simulink library "Utilities"  (R2020b)
settings: Solver=VariableStepAuto  StartTime=0.0  StopTime=10.0  RelTol=1e-3

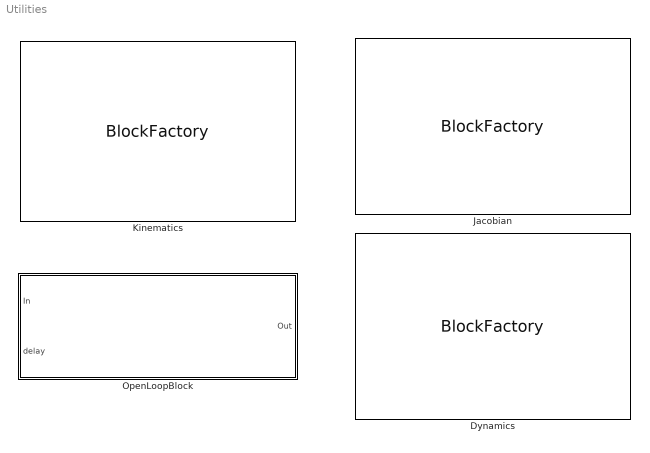
== system Utilities ==
  Dynamics : S-Function  FunctionName=BlockFactory  Parameters='XBotBlock_Dynamics','Dynamics',ModelName,ComponentsList  SFunctionDeploymentMode=off  EnableBusSupport=off  mask{ModelName=DefaultModel, ComponentsList={ 'B', 'BInv', 'M', 'H', 'tau_g', 'tau_id', 'tau_id_const' }}
  Jacobian : S-Function  FunctionName=BlockFactory  Parameters='XBotBlock_Jacobian','Jacobian',ModelName,JacobianList,LinkName,TargetFrame,ExternalRef,TargetLink,BaseLink  SFunctionDeploymentMode=off  EnableBusSupport=off  mask{ModelName=DefaultModel, JacobianList={ 'J', 'J_postural', 'J_relative', 'J_COM', 'dJcomQdot', 'JdotQdot', 'JdotQdot_relative' }, LinkName=, TargetFrame=, ExternalRef=Off, TargetLink=, BaseLink=}
      mask init:
      | mask_params = Simulink.Mask.get(gcb);
      | link_frame_param= mask_params.Parameters(3);
      | target_frame_param = mask_params.Parameters(4);
      | ext_ref_param = mask_params.Parameters(5);
      | target_link_param= mask_params.Parameters(6);
      | base_link_param = mask_params.Parameters(7);
      | 
      | 
      | set_enabled=false;
      | if(~bdIsLibrary(bdroot))
      |     model_status=get_param(bdroot,'SimulationStatus');
      |     if(model_status=="stopped")
      |         set_enabled=true;
      |     end
      | else
      |     set_enabled=true;
      | end
      | 
      | if(set_enabled)
      |     link_frame_param.set('Enabled','off'); 
      |     target_frame_param.set('Enabled','off');  
      |     ext_ref_param.set('Enabled','off');  
      |     target_link_param.set('Enabled','off');   
      |     base_link_param.set('Enabled','off');   
      | 
      | 
      |     %Get Number of input and output ports.
      |     portHandles = get_param(gcb,'PortHandles');
      |     %Input ports
      |     inputPorts=length(portHandles.Inport);
      |     %Output ports
      |     outputPorts=length(portHandles.Outport);
      | 
      | 
      |     % Get block mask handle
      |     maskObj = Simulink.Mask.get(gcb); 
      | 
      |     % Readings Selected
      |     itemsSelected=maskObj.getParameter('JacobianList').Value;
      |     itemsSelected=regexprep(itemsSelected,'[^a-zA-Z0-9,_]','');
      |     itemsSplitted=split(itemsSelected,',');
      | 
      |     external_ref=get_param(gcb, 'ExternalRef');
      |     for index=1:length(itemsSplitted)
      |         item=itemsSplitted{index};
      |         if(item=="J")
      |             link_frame_param.set('Enabled','on'); 
      |             ext_ref_param.set('Enabled','on');
      |             if(external_ref ~="On")
      |                 target_frame_param.set('Enabled','on'); 
      |             end
      |         end
      |         if(item=="J_relative" || item=="JdotQdot_relative")
      |             target_link_param.set('Enabled','on');   
      |             base_link_param.set('Enabled','on');   
      |         end
      |     end
      | end
  Kinematics : S-Function  FunctionName=BlockFactory  Parameters='XBotBlock_Kinematics','Kinematics',ModelName,PoseList,SourceFrame,TargetFrame,TwistList,LinkName,BaseLinkName,COMList,ReferenceFrame  SFunctionDeploymentMode=off  EnableBusSupport=off  mask{ModelName=DefaultModel, PoseList={ 'Pose' }, SourceFrame=, TargetFrame=, LinkNamePose=, TwistList={ 'v_tw', 'a_tw' }, LinkName=, BaseLinkName=, COMList={ 'p_COM', 'v_COM', 'a_COM' }, ReferenceFrame=}
      mask prompts: LinkNamePose "LinkName"
      mask init:
      | % Get block mask handle
      | maskObj = Simulink.Mask.get(gcb); 
      | 
      | % Pose Selected
      | itemsSelected=maskObj.getParameter('PoseList').Value;
      | itemsSelected=regexprep(itemsSelected,'[^a-zA-Z0-9,_]','');
      | itemsSplitted=split(itemsSelected,',');
      | 
      | point_acc_prensence=0;
      | for index=1:length(itemsSplitted)
      |     item=itemsSplitted{index};
      |     if(~isempty(item));
      |         if(item=="PointAcc")
      |             point_acc_prensence=1;
      |         end
      |     end
      | end
      | 
      | if(point_acc_prensence==0)
      |     link_name=get_param(gcb, 'LinkName');
      |     set_param(gcb,'LinkNamePose',link_name);
      | else
      |    link_name_pose=get_param(gcb, 'LinkNamePose');
      |    set_param(gcb,'LinkName',link_name_pose);
      | end
  OpenLoopBlock : Subsystem

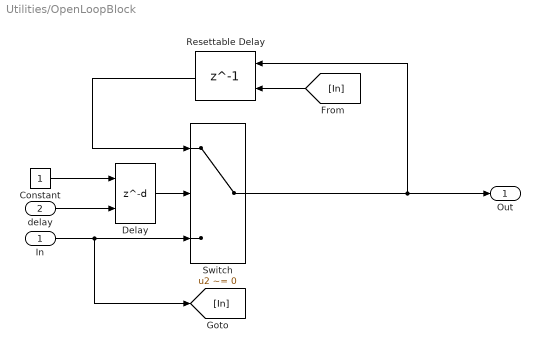
== system Utilities/OpenLoopBlock ==
  In : Inport
  delay : Inport  Port=2
  Constant : Constant
  Delay : Delay  DelayLengthSource=Input port  DelayLength=1  InitialCondition=0
  Resettable Delay : Delay  DelayLength=1  InitialConditionSource=Input port
  Switch : Switch  Criteria=u2 ~= 0
  Out : Outport
  wires:
  Delay/1 -> Switch/2
  Constant/1 -> Delay/1
  In/1 -> [In], Switch/3
  Switch/1 -> Out/1, Resettable Delay/1
  Resettable Delay/1 -> Switch/1
  [In] -> Resettable Delay/2
  delay/1 -> Delay/2
